simulink model "sim5"  (R2013a)
settings: Solver=ode45  StartTime=0.0  StopTime=10  RelTol=1e-3
values from neighbouring files (symbols this model uses):
  a = [ (5*Twewn - 4*Tzewn - Tpn), 0; (Twewn - Tpn), (-4)*(Tpn-Tzewn)]    [skrypt2.m]    (also in skrypt5.m = 1)
  czas_skoku = 0    [skrypt4.m]    (also in skrypt5.m = 2)
  d = 1    [skrypt5.m]
  d1u = 0    [skrypt5.m]
  dt = 0.05    [skrypt5.m]
  du = 0')    [skrypt4.m]    (also in skrypt5.m = 0)
  ksi = tabksi(i)    [skrypt5.m]
  u0 = 0    [skrypt4.m]    (also in skrypt5.m = 1)
  u10 = 0    [skrypt5.m]
  w = 3    [skrypt5.m]
  x0 = (-10/3)+b*u0/a0    (= -3.33333333333)    [skrypt4.m]    (also in skrypt5.m = tabx0(k))
  x10 = tabx10(j)    [skrypt5.m]
settings Model: Creator=LAB320-1552  LastModifiedBy=Dawidek

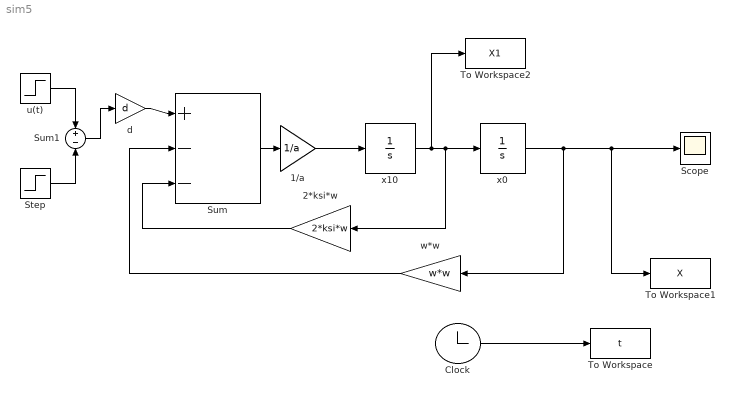
== system sim5 ==
  1/a : Gain  Gain=1/a
  2*ksi*w : Gain  Gain=2*ksi*w
  Clock : Clock
  Scope : Scope
  Step : Step  Time=czas_skoku + dt  Before=u10  After=u10+d1u  SampleTime=dt
  Sum : Sum  Inputs=+|-|-
  Sum1 : Sum  Inputs=+-
  To Workspace : ToWorkspace  VariableName=t  SampleTime=-1
  To Workspace1 : ToWorkspace  VariableName=X  SampleTime=-1
  To Workspace2 : ToWorkspace  VariableName=X1  SampleTime=-1
  d : Gain  Gain=d
  u(t) : Step  Time=czas_skoku  Before=u0  After=u0+du  SampleTime=dt
  w*w : Gain  Gain=w*w
  x0 : Integrator  InitialCondition=x0
  x10 : Integrator  InitialCondition=x10
  wires:
  d/1 -> Sum/1
  Sum/1 -> 1/a/1
  1/a/1 -> x10/1
  x10/1 -> x0/1, 2*ksi*w/1, To Workspace2/1
  2*ksi*w/1 -> Sum/3
  x0/1 -> w*w/1, To Workspace1/1, Scope/1
  w*w/1 -> Sum/2
  Clock/1 -> To Workspace/1
  Step/1 -> Sum1/2
  Sum1/1 -> d/1
  u(t)/1 -> Sum1/1
